simulink model "PP_TDPA_TD"  (R2021b)
settings: Solver=FixedStepAuto  StartTime=0.0  StopTime=20  FixedStep=0.001  RelTol=1e-3
settings Model: Creator=lucao  LastModifiedBy=lucao

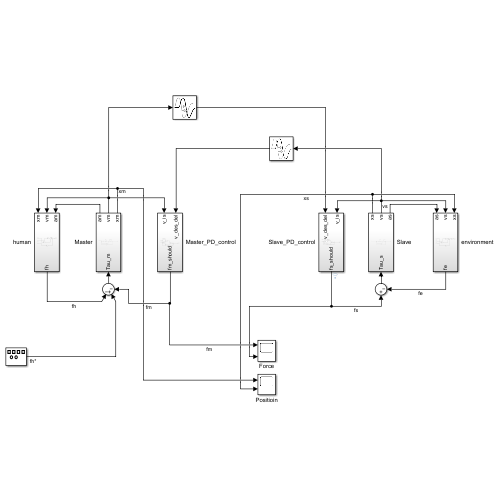
[thumbnail: Simulink's stored preview of the top-level diagram]
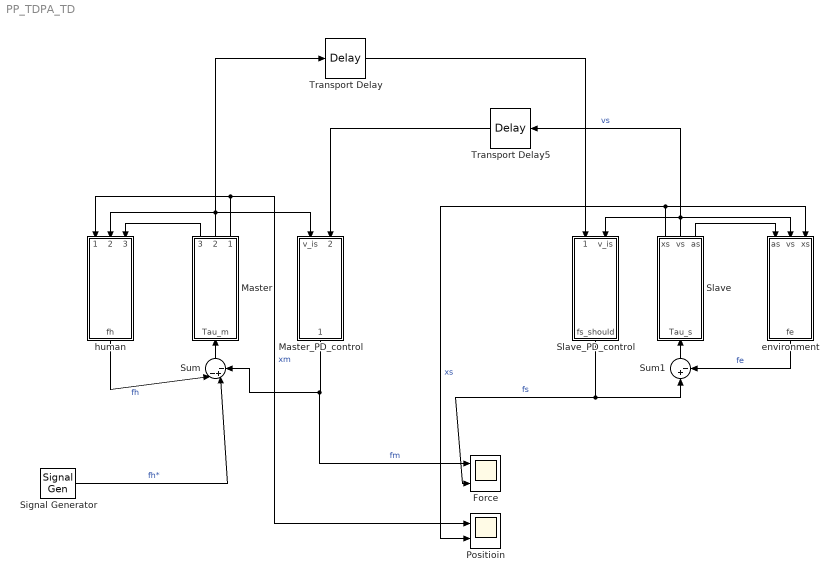
== system PP_TDPA_TD ==
  Force : Scope  NumInputPorts=2
  Master : Subsystem
  Master_PD_control : Subsystem
  Positioin : Scope  NumInputPorts=2
  Signal Generator : SignalGenerator  Amplitude=10  Frequency=0.5
  Slave : Subsystem
  Slave_PD_control : Subsystem
  Sum : Sum  Inputs=|-+-
  Sum1 : Sum  Inputs=|+-
  Transport Delay : TransportDelay  DelayTime=0
  Transport Delay5 : TransportDelay  DelayTime=0
  environment : Subsystem
  human : Subsystem
  wires:
  human/1(fh) -> Sum/1  "fh"
  Sum/1 -> Master/1(Tau_m)
  Master_PD_control/1(fm_should) -> Force/1, Sum/3  "fm"
  Sum1/1 -> Slave/1(Tau_s)
  environment/1(fe) -> Sum1/2  "fe"
  Slave_PD_control/1(fs_should) -> Sum1/1, Force/2  "fs"
  Master/1(xm) -> human/1(xm), Positioin/1  "xm"
  Slave/1(xs) -> Positioin/2, environment/3(xs)  "xs"
  Signal Generator/1 -> Sum/2  "fh*"
  Master/3(am) -> human/3(am)
  Master/2(vm) -> Transport Delay/1, Master_PD_control/1(v_is), human/2(vm)
  Slave/3(as) -> environment/1(as)
  Slave/2(vs) -> Slave_PD_control/2(v_is), Transport Delay5/1, environment/2(vs)  "vs"
  Transport Delay/1 -> Slave_PD_control/1(v_des_del)
  Transport Delay5/1 -> Master_PD_control/2(v_des_del)

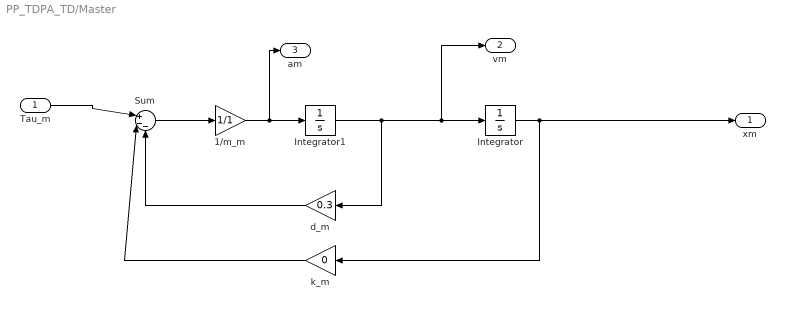
== system PP_TDPA_TD/Master ==
  Tau_m : Inport
  1/m_m : Gain  Gain=1/1
  Integrator : Integrator
  Integrator1 : Integrator
  Sum : Sum  Inputs=|+--
  d_m : Gain  Gain=0.3
  k_m : Gain  Gain=0
  xm : Outport
  vm : Outport  Port=2
  am : Outport  Port=3
  wires:
  Integrator/1 -> k_m/1, xm/1
  Integrator1/1 -> d_m/1, vm/1, Integrator/1
  Tau_m/1 -> Sum/1
  d_m/1 -> Sum/3
  k_m/1 -> Sum/2
  Sum/1 -> 1/m_m/1
  1/m_m/1 -> am/1, Integrator1/1

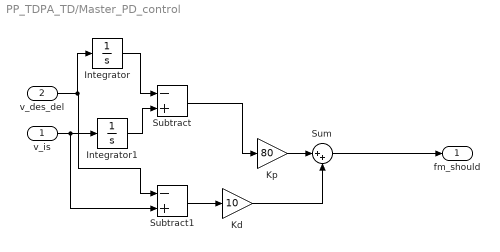
== system PP_TDPA_TD/Master_PD_control ==
  v_is : Inport
  v_des_del : Inport  Port=2
  Integrator : Integrator
  Integrator1 : Integrator
  Kd : Gain  Gain=10
  Kp : Gain  Gain=80
  Subtract : Sum  Inputs=-+
  Subtract1 : Sum  Inputs=-+
  Sum : Sum  Inputs=|++
  fm_should : Outport
  wires:
  Subtract/1 -> Kp/1
  Subtract1/1 -> Kd/1
  Kp/1 -> Sum/1
  Kd/1 -> Sum/2
  Sum/1 -> fm_should/1
  v_des_del/1 -> Subtract1/1, Integrator/1
  v_is/1 -> Subtract1/2, Integrator1/1
  Integrator/1 -> Subtract/1
  Integrator1/1 -> Subtract/2

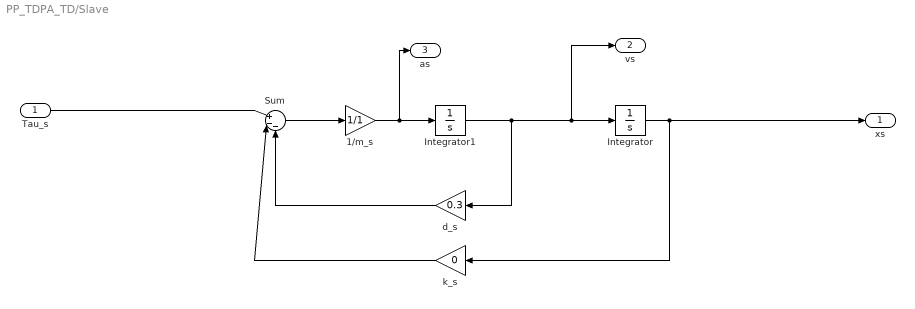
== system PP_TDPA_TD/Slave ==
  Tau_s : Inport
  1/m_s : Gain  Gain=1/1
  Integrator : Integrator
  Integrator1 : Integrator
  Sum : Sum  Inputs=|+--
  d_s : Gain  Gain=0.3
  k_s : Gain  Gain=0
  xs : Outport
  vs : Outport  Port=2
  as : Outport  Port=3
  wires:
  Integrator/1 -> k_s/1, xs/1
  Integrator1/1 -> d_s/1, vs/1, Integrator/1
  Tau_s/1 -> Sum/1
  d_s/1 -> Sum/3
  k_s/1 -> Sum/2
  Sum/1 -> 1/m_s/1
  1/m_s/1 -> as/1, Integrator1/1

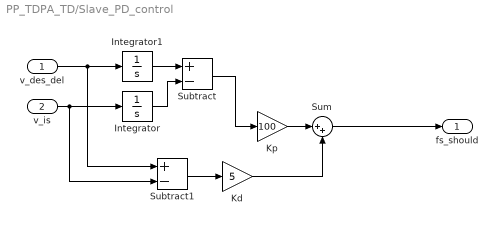
== system PP_TDPA_TD/Slave_PD_control ==
  v_des_del : Inport
  v_is : Inport  Port=2
  Integrator : Integrator
  Integrator1 : Integrator
  Kd : Gain  Gain=5
  Kp : Gain  Gain=100
  Subtract : Sum  Inputs=+-
  Subtract1 : Sum  Inputs=+-
  Sum : Sum  Inputs=|++
  fs_should : Outport
  wires:
  v_des_del/1 -> Integrator1/1, Subtract1/1
  v_is/1 -> Subtract1/2, Integrator/1
  Subtract/1 -> Kp/1
  Subtract1/1 -> Kd/1
  Kp/1 -> Sum/1
  Kd/1 -> Sum/2
  Sum/1 -> fs_should/1
  Integrator/1 -> Subtract/2
  Integrator1/1 -> Subtract/1

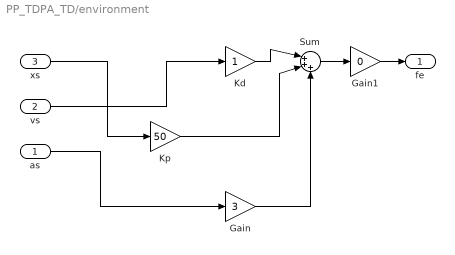
== system PP_TDPA_TD/environment ==
  as : Inport
  vs : Inport  Port=2
  xs : Inport  Port=3
  Gain : Gain  Gain=3
  Gain1 : Gain  Gain=0
  Kd : Gain
  Kp : Gain  Gain=50
  Sum : Sum  Inputs=|+++
  fe : Outport
  wires:
  xs/1 -> Kp/1
  vs/1 -> Kd/1
  Kp/1 -> Sum/2
  Kd/1 -> Sum/1
  Sum/1 -> Gain1/1
  as/1 -> Gain/1
  Gain/1 -> Sum/3
  Gain1/1 -> fe/1

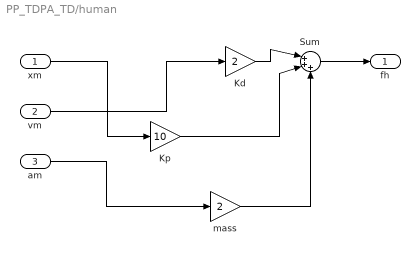
== system PP_TDPA_TD/human ==
  xm : Inport
  vm : Inport  Port=2
  am : Inport  Port=3
  Kd : Gain  Gain=2
  Kp : Gain  Gain=10
  Sum : Sum  Inputs=|+++
  mass : Gain  Gain=2
  fh : Outport
  wires:
  vm/1 -> Kd/1
  Kp/1 -> Sum/2
  Kd/1 -> Sum/1
  Sum/1 -> fh/1
  xm/1 -> Kp/1
  am/1 -> mass/1
  mass/1 -> Sum/3
